simulink model "GFLIB_Acos_BAM_FLT"  (Simulink 8.3)
settings: Solver=ode45  StartTime=0.0  StopTime=10.0  RelTol=1e-3
settings Model: Creator=B37097  LastModifiedBy=B17364
settings DataIOCC: SignalLoggingSaveFormat=Dataset
settings DebuggingCC: UnderspecifiedInitializationDetection=Simplified  StateNameClashWarn=none
settings GRTTargetCC: CombineOutputUpdateFcns=on  GRTInterface=off

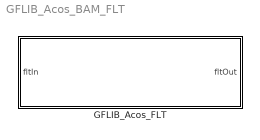
== system GFLIB_Acos_BAM_FLT ==
  GFLIB_Acos_FLT : Subsystem  mask(GFLIB_Acos_FLT){}
      mask help: Bit accurate model of GFLIB_Acos function, which computes the acos(fltIn) using the square based approximation.
      mask init:
      | pos = get_param(gcb, 'Position');width = pos(3) - pos(1); height = pos(4) - pos(2);tX=width/2;tY=height*0.9;
      mask Display: color('black');port_label('input',1,'fltIn');port_label('output',1,'fltOut');color('black');disp('GFLIB_Acos_FLT');color('blue');text(tX,tY, 'BAM', 'horizontalAlignment', 'center');

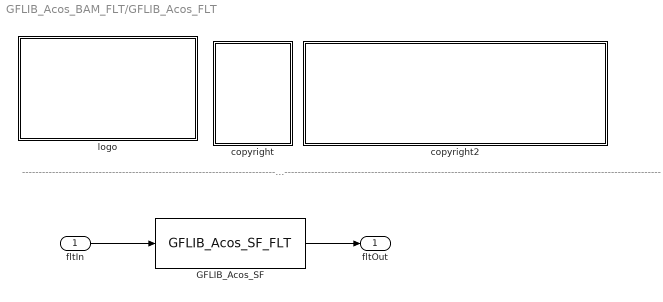
== system GFLIB_Acos_BAM_FLT/GFLIB_Acos_FLT ==
  note: ---------------------------------------------------------------------------------------------------------------------------------------------------------------------------------------------------
  fltIn : Inport
  GFLIB_Acos_SF : S-Function  FunctionName=GFLIB_Acos_SF_FLT  EnableBusSupport=off
  copyright : Subsystem
      mask Display:
      | text(10,90,'FILE:');text(10,75,'DESRIPTION:')
      | text(10,60,'COPYRIGHT:')
      | text(10,45,'VERSION:')
      | text(10,30,'DATE:')
  copyright2 : Subsystem
      mask Display:
      | text(10,90,'GFLIB_Acos_BAM_FLT.mdl');text(10,75,'Inverse cosine transformation');text(10,60,'Freescale')
      | text(10,45,'0.1');text(10,30,'31-Aug-2011');
  logo : Subsystem
      mask Display: image(imread('logo.jpg'))
  fltOut : Outport
  wires:
  fltIn/1 -> GFLIB_Acos_SF/1
  GFLIB_Acos_SF/1 -> fltOut/1

== system GFLIB_Acos_BAM_FLT/GFLIB_Acos_FLT/copyright ==

== system GFLIB_Acos_BAM_FLT/GFLIB_Acos_FLT/copyright2 ==

== system GFLIB_Acos_BAM_FLT/GFLIB_Acos_FLT/logo ==
